simulink model "wecs"  (Simulink 8.7)
settings: Solver=VariableStepAuto  StartTime=0.0  StopTime=10.0  FixedStep=10e-6  RelTol=1e-3
undefined symbols (not defined in the file): DiscIntNeverNeededParam
libraries: powerlib x7, powerlib_meascontrol x2, simulink x1, re_lib x1
settings Model: Creator=GNEX  LastModifiedBy=ikuma
settings DataIOCC: LimitDataPoints=off  SaveFormat=Dataset
settings DebuggingCC: UnderspecifiedInitializationDetection=Simplified  MergeDetectMultiDrivingBlocksExec=error
settings HardwareCC: ProdBitPerPointer=64  ProdLargestAtomicFloat=Float  ProdIntDivRoundTo=Zero  ProdEndianess=LittleEndian  ProdWordSize=64  ProdHWDeviceType=Intel->x86-64 (Windows64)
settings ModelReferenceCC: PropagateSignalLabelsOutOfModel=on
settings ConfigComp: CovModelRefEnable=off

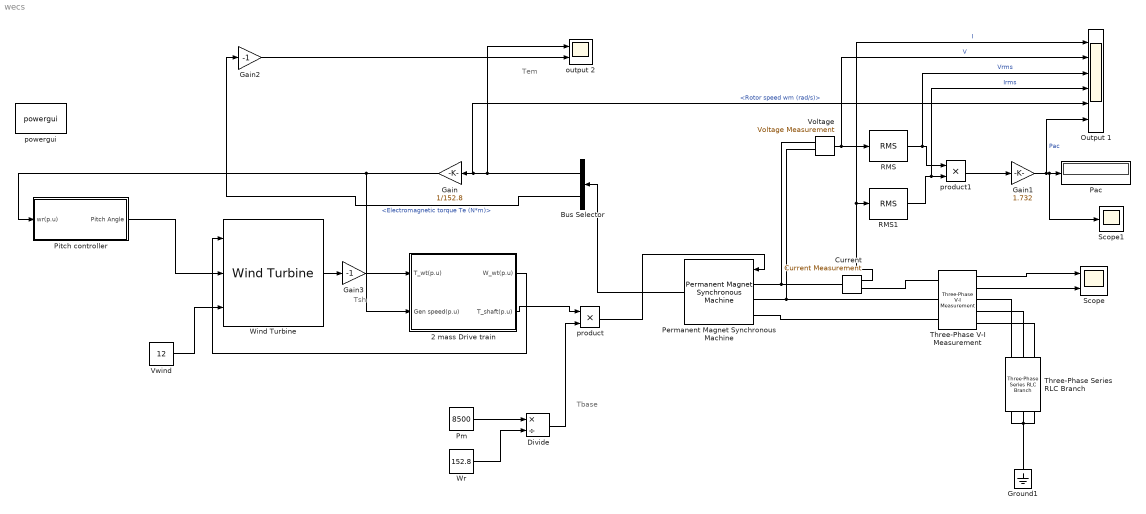
== system wecs ==
  note: Tem
  note: Tbase
  note: Tsh
  2 mass Drive train : Subsystem
  Bus Selector : BusSelector  OutputSignals=Rotor speed wm (rad/s),Electromagnetic torque Te (N*m)
  "Current " : powerlib/Measurements/Current Measurement  PhasorSimulation=off  OutputType=Complex  PSBequivalent=0
  Divide : Product  Inputs=*/
  Gain : Gain  Gain=1/152.8
  Gain1 : Gain  Gain=1.732
  Gain2 : Gain  Gain=-1
  Gain3 : Gain  Gain=-1
  Ground1 : powerlib/Elements/Ground  LConnTagsString=a
  Output 1 : Scope  NumInputPorts=6
  Pac : Display
  Permanent Magnet Synchronous Machine : powerlib/Machines/Permanent Magnet Synchronous Machine  NbPhases=3  FluxDistribution=Sinusoidal  RotorType=Round  MechanicalLoad=Torque Tm  PresetModel=No  ShowDetailedParameters=on  MeasurementBus=off  Resistance=0.0425  Inductance=8.5e-3  dqInductances=[8.5e-3,8.5e-3]  La=0.000395  MachineConstant=Flux linkage established by magnets (V.s)  Flux=0.433  VoltageCst=392.6876  TorqueCst=3.2475  Flat=120  Mechanical=[0.01197 0.001189 5 0]  PolePairs=4  InitialConditions=[0,0, 0,0]  InitialConditions5ph=[0 0 0 0 0 0]  TsPowergui=0  TsBlock=-1  RefAngle=90 degrees behind phase A axis (modified Park)
  Pitch controller : Subsystem
  Pm : Constant  Value=8500
  RMS : powerlib_meascontrol/Measurements/RMS  TrueRMS=on  Freq=50  RMSInit=120  Ts=50e-6
  RMS1 : powerlib_meascontrol/Measurements/RMS  TrueRMS=on  Freq=50  RMSInit=120  Ts=50e-6
  Scope : Scope  NumInputPorts=2
  Scope1 : Scope
  Three-Phase Series RLC Branch : powerlib/Elements/Three-Phase Series RLC Branch  LConnTagsString=A|B|C  RConnTagsString=A|B|C  BranchType=R  Resistance=25  Inductance=1e-3  Capacitance=1e-6  Measurements=None
  Three-Phase V-I Measurement : powerlib/Measurements/Three-Phase V-I Measurement  VoltageMeasurement=phase-to-phase  SetLabelV=off  LabelV=Vabc  Vpu=off  VpuLL=off  CurrentMeasurement=yes  SetLabelI=off  LabelI=Iabc  Ipu=off  Pbase=100e6  Vbase=500e3  OutputType=Complex  PhasorSimulation=off  PSBequivalent=0
  "Voltage " : powerlib/Measurements/Voltage Measurement  PhasorSimulation=off  OutputType=Complex  PSBequivalent=0
  Vwind : Constant  Value=12
  Wind Turbine : re_lib/Wind Generation/Wind Turbine  Pnom=8.5e3  Pelec_base=8.5e3/0.9  wind_base=12  P_wind_base=0.8  speed_nom=1  pitch_angle=0  c1_c6="[0.51763          116          0.4            5           21     0.006795]"  cp_nom=0.48  lambda_nom=8.1
  Wr : Constant  Value=152.8
  "output 2 " : Scope  NumInputPorts=2
  powergui : powerlib/powergui  Priority=1  SimulationMode=Discrete  SolverType=Tustin/Backward Euler (TBE)  SampleTime=20e-6  frequency=60  SPID=off  DisableSnubberDevices=off  DisableRonSwitches=off  DisableVfSwitches=off  SwTol=0  DisplayEquations=off  Interpol=off  ExternalGateDelay=off  methode=off  Ts=10  FunctionMessages=off  echomessages=off  HookPort=off  EnableUseOfTLC=off  x0status=blocks  frequencyindice=0  Pbase=100e6  ErrMax=1e-4  Iterations=50  UnitsV=kV  UnitsW=MW  buscounter=0  RestoreLinks=warning  ResistiveCurrentMeasurement=off  Frange=[0:2:500]  Ylog=off  Xlog=on  ShowGrid=off  save=off  variable=ZData  structure=0  ZoomFFT=off  StartTime=0.0  cycles=1  DisplayStyle=1  fundamental=60  FreqAxis=off  MaxFrequency=1000  frequencyindicesteady=1  RmsSteady=1  display=off
  product : Product
  product1 : Product
  wires:
  Pitch controller/1("Pitch Angle ") -> Wind Turbine/2
  Vwind/1 -> Wind Turbine/3
  Permanent Magnet Synchronous Machine/1 -> Bus Selector/1
  Bus Selector/1 -> "output 2 "/1, Output 1/5, Gain/1  "<Rotor speed wm (rad/s)>"
  Gain/1 -> 2 mass Drive train/2(Gen speed(p.u)), Pitch controller/1(wr(p.u))
  2 mass Drive train/1(W_wt(p.u)) -> Wind Turbine/1
  2 mass Drive train/2(T_shaft(p.u)) -> product/1
  Pm/1 -> Divide/1
  Wr/1 -> Divide/2
  Divide/1 -> product/2
  product/1 -> Permanent Magnet Synchronous Machine/1
  Three-Phase V-I Measurement/1 -> Scope/1
  Three-Phase V-I Measurement/2 -> Scope/2
  "Current "/1 -> Output 1/1, RMS1/1  "I"
  RMS/1 -> Output 1/3, product1/1  "Vrms"
  RMS1/1 -> Output 1/4, product1/2  "Irms"
  product1/1 -> Gain1/1
  Gain1/1 -> Output 1/6, Scope1/1, Pac/1  "Pac"
  "Voltage "/1 -> Output 1/2, RMS/1  "V"
  Bus Selector/2 -> Gain2/1  "<Electromagnetic torque Te (N*m)>"
  Wind Turbine/1 -> Gain3/1
  Gain3/1 -> 2 mass Drive train/1(T_wt(p.u))
  Gain2/1 -> "output 2 "/2
  connections:
  Three-Phase Series RLC Branch/RConn1 -- Three-Phase Series RLC Branch/RConn3 -- Ground1/LConn1 -- Three-Phase Series RLC Branch/RConn2
  Permanent Magnet Synchronous Machine/LConn1 -- "Current "/LConn1 -- "Voltage "/LConn1
  Permanent Magnet Synchronous Machine/LConn2 -- Three-Phase V-I Measurement/LConn2 -- "Voltage "/LConn2
  Permanent Magnet Synchronous Machine/LConn3 -- Three-Phase V-I Measurement/LConn3
  Three-Phase V-I Measurement/RConn1 -- Three-Phase Series RLC Branch/LConn1
  Three-Phase V-I Measurement/RConn2 -- Three-Phase Series RLC Branch/LConn2
  Three-Phase V-I Measurement/RConn3 -- Three-Phase Series RLC Branch/LConn3
  "Current "/RConn1 -- Three-Phase V-I Measurement/LConn1

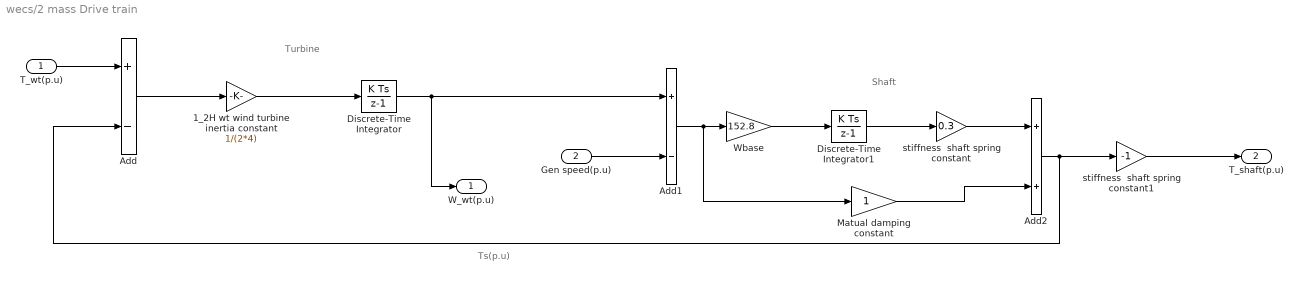
== system wecs/2 mass Drive train ==
  note: Shaft
  note: Turbine
  note: Ts(p.u)
  T_wt(p.u) : Inport
  Gen speed(p.u) : Inport  Port=2
  1_2H wt wind turbine inertia constant : Gain  Gain=1/(2*4)
  Add : Sum  Inputs=+-
  Add1 : Sum  Inputs=+-
  Add2 : Sum
  Discrete-Time Integrator : DiscreteIntegrator  InitialCondition=1  InitialConditionSetting=State (most efficient)  SampleTime=50e-6  ICPrevOutput=DiscIntNeverNeededParam  ICPrevScaledInput=DiscIntNeverNeededParam
  Discrete-Time Integrator1 : DiscreteIntegrator  InitialCondition=1/0.3  InitialConditionSetting=State (most efficient)  SampleTime=50e-6  ICPrevOutput=DiscIntNeverNeededParam  ICPrevScaledInput=DiscIntNeverNeededParam
  Matual damping constant : Gain
  Wbase : Gain  Gain=152.8
  stiffness  shaft spring constant : Gain  Gain=0.3
  stiffness  shaft spring constant1 : Gain  Gain=-1
  W_wt(p.u) : Outport
  T_shaft(p.u) : Outport  Port=2
  wires:
  T_wt(p.u)/1 -> Add/1
  Add/1 -> 1_2H wt wind turbine inertia constant/1
  1_2H wt wind turbine inertia constant/1 -> Discrete-Time Integrator/1
  Discrete-Time Integrator/1 -> W_wt(p.u)/1, Add1/1
  Gen speed(p.u)/1 -> Add1/2
  Add1/1 -> Matual damping constant/1, Wbase/1
  Wbase/1 -> Discrete-Time Integrator1/1
  Discrete-Time Integrator1/1 -> stiffness  shaft spring constant/1
  stiffness  shaft spring constant/1 -> Add2/1
  Matual damping constant/1 -> Add2/2
  Add2/1 -> Add/2, stiffness  shaft spring constant1/1
  stiffness  shaft spring constant1/1 -> T_shaft(p.u)/1

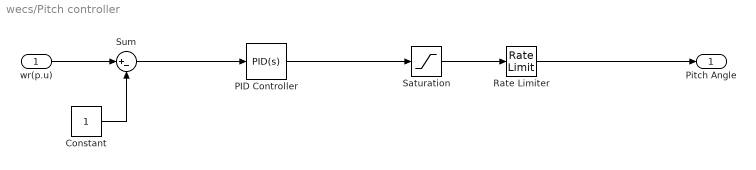
== system wecs/Pitch controller ==
  wr(p.u) : Inport
  Constant : Constant
  PID Controller : simulink/Continuous/PID Controller  Controller=PID  TimeDomain=Continuous-time  SampleTime=-1  IntegratorMethod=Forward Euler  FilterMethod=Forward Euler  Form=Parallel  UseFilter=on  ControllerParametersSource=internal  P=40.5  I=15.09  D=-6.612  N=0.568  InitialConditionSource=internal  InitialConditionForIntegrator=0  InitialConditionForFilter=0  ExternalReset=none  LimitOutput=off  UpperSaturationLimit=inf  LowerSaturationLimit=-inf  LinearizeAsGain=on  AntiWindupMode=none  Kb=1  TrackingMode=off  Kt=1  PParamMin=[]  PParamMax=[]  IParamMin=[]  IParamMax=[]  DParamMin=[]  DParamMax=[]  NParamMin=[]  NParamMax=[]  KbParamMin=[]  KbParamMax=[]  KtParamMin=[]  KtParamMax=[]  POutMin=[]  POutMax=[]  IOutMin=[]  IOutMax=[]  DOutMin=[]  DOutMax=[]  NOutMin=[]  NOutMax=[]  KbOutMin=[]  KbOutMax=[]  KtOutMin=[]  KtOutMax=[]  IntegratorOutMin=[]  IntegratorOutMax=[]  FilterOutMin=[]  FilterOutMax=[]  SumOutMin=[]  SumOutMax=[]  SumI1OutMin=[]  SumI1OutMax=[]  SumI2OutMin=[]  SumI2OutMax=[]  SumI3OutMin=[]  SumI3OutMax=[]  SumDOutMin=[]  SumDOutMax=[]  SaturationOutMin=[]  SaturationOutMax=[]  IntegratorContinuousStateAttributes=''  IntegratorStateMustResolveToSignalObject=off  IntegratorRTWStateStorageClass=Auto  FilterContinuousStateAttributes=''  FilterStateMustResolveToSignalObject=off  FilterRTWStateStorageClass=Auto  DifferentiatorICPrevScaledInput=0  DifferentiatorOutMin=[]  DifferentiatorOutMax=[]
  Rate Limiter : RateLimiter  RisingSlewLimit=2  FallingSlewLimit=-2  SampleTimeMode=inherited
  Saturation : Saturate  UpperLimit=45  LowerLimit=0
  Sum : Sum  Inputs=|+-
  "Pitch Angle " : Outport
  wires:
  wr(p.u)/1 -> Sum/1
  Constant/1 -> Sum/2
  Sum/1 -> PID Controller/1
  Saturation/1 -> Rate Limiter/1
  Rate Limiter/1 -> "Pitch Angle "/1
  PID Controller/1 -> Saturation/1
